simulink model "FrequencyMeasurement"  (R2021a)
settings: Solver=VariableStepDiscrete  StartTime=0.0  StopTime=10.0  MaxStep=5e-4  RelTol=1e-3
settings Model: Creator=Sajid Ali  LastModifiedBy=Sajid Ali

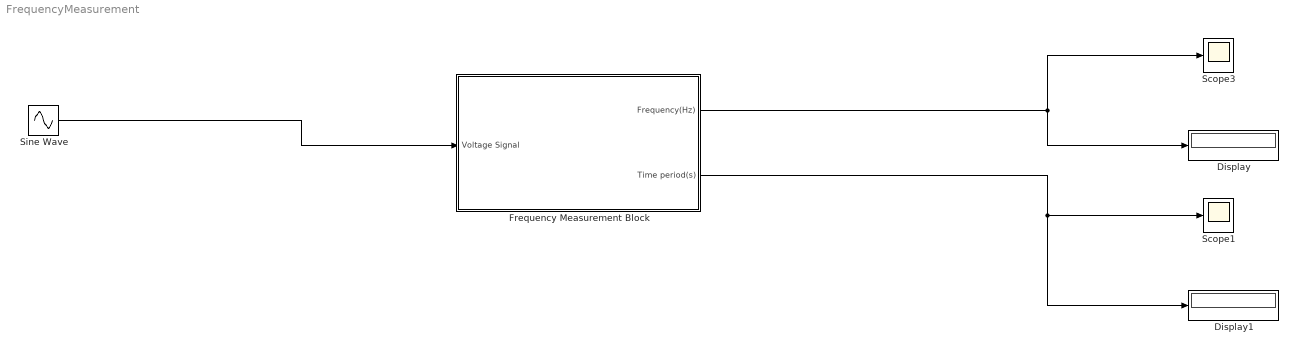
== system FrequencyMeasurement ==
  Display : Display
  Display1 : Display
  Frequency Measurement Block : Subsystem  mask(Frequency measurement by zero Corssing){MinimumFrequncy=47, MaximumFrequency=55}
      mask prompts: MinimumFrequncy "Minimum Frequency (Hz)"; MaximumFrequency "Maximum Frequency (Hz)"
      mask help:
      | This block measures the frquency by zero crossing method. To get accurate Results use fixed step simulation mode.
      | author:
      | Sajid Ali
      | sajid.ali@skyelectric.com
      mask Display: image('C:\Users\Sajid Ali\Pictures\Frequency measurement2.PNG'); % Use "Edit Image" on toolstrip to change.
  Scope1 : Scope
  Scope3 : Scope
  Sine Wave : Sin  Frequency=2*pi*49.01  SampleTime=0
  wires:
  Frequency Measurement Block/1(Frequency(Hz)) -> Scope3/1, Display/1
  Sine Wave/1 -> Frequency Measurement Block/1(Voltage Signal)
  Frequency Measurement Block/2(Time period(s)) -> Display1/1, Scope1/1

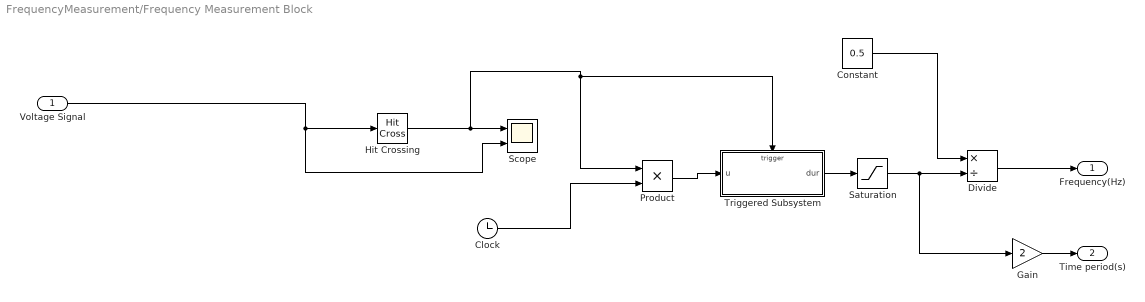
== system FrequencyMeasurement/Frequency Measurement Block ==
  Voltage Signal : Inport
  Clock : Clock
  Constant : Constant  Value=0.5
  Divide : Product  Inputs=*/
  Gain : Gain  Gain=2
  Hit Crossing : HitCross
  Product : Product
  Saturation : Saturate  UpperLimit=1/MinimumFrequncy/2  LowerLimit=1/MaximumFrequency/2
  Scope : Scope  NumInputPorts=2
  Triggered Subsystem : Subsystem  TreatAsAtomicUnit=on
  Frequency(Hz) : Outport
  Time period(s) : Outport  Port=2
  wires:
  Hit Crossing/1 -> Triggered Subsystem/Trigger, Product/1, Scope/1
  Voltage Signal/1 -> Scope/2, Hit Crossing/1
  Saturation/1 -> Gain/1, Divide/2
  Product/1 -> Triggered Subsystem/1(u)
  Triggered Subsystem/1(dur) -> Saturation/1
  Clock/1 -> Product/2
  Constant/1 -> Divide/1
  Divide/1 -> Frequency(Hz)/1
  Gain/1 -> Time period(s)/1

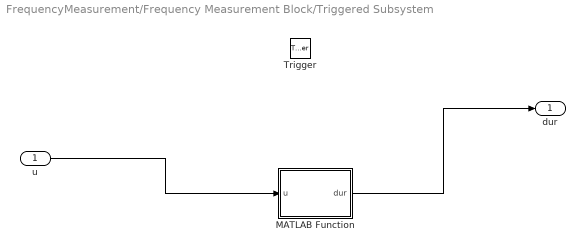
== system FrequencyMeasurement/Frequency Measurement Block/Triggered Subsystem ==
  u : Inport
  Trigger : TriggerPort  VariantControl=(inherit)
  MATLAB Function : MATLAB Function  TreatAsAtomicUnit=on
  dur : Outport
  wires:
  u/1 -> MATLAB Function/1(u)
  MATLAB Function/1(dur) -> dur/1

== matlab function FrequencyMeasurement/Frequency Measurement Block/Triggered Subsystem/MATLAB Function ==
  data: u input; dur output
function dur = fcn(u)
persistent prev;
if isempty(prev)
    prev=0;
end
if (u~=0)
    dur=u-prev;
    prev=u;
else
    dur=0;
end
